simulink model "ex2"  (R2021a)
settings: Solver=VariableStepAuto  StartTime=0.0  StopTime=10.0  RelTol=1e-3
undefined symbols (not defined in the file or in its folder): B, g, I_xx, I_yy, I_zz, k, kd, l, m
settings Model: Creator=frede  LastModifiedBy=frede
settings DataIOCC: ReturnWorkspaceOutputs=off

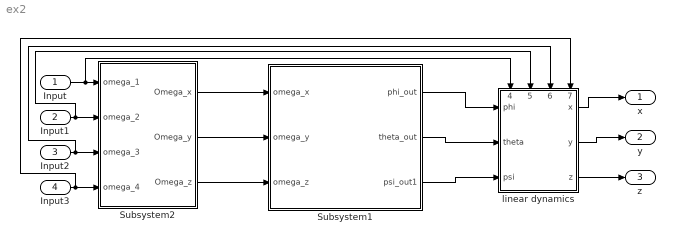
== system ex2 ==
  Input : Inport
  Input1 : Inport  Port=2
  Input2 : Inport  Port=3
  Input3 : Inport  Port=4
  Subsystem1 : Subsystem
  Subsystem2 : Subsystem
  linear dynamics : Subsystem
      settings: PortSchema="{\"entries\":[{\"content\":{\"sides\":[{\"content\":{\"connectorIds\":[\"In1\",\"In2\",\"In3\"]},\"type\":\"ConnectorPlacement.EquallySpacedRectSide\",\"uuid\":\"56efaa7c-52a2-4b92-9bf3-e77850251265\"},{\"content\":{\"connectorIds\":[\"Out1\",\"Out2\",\"Out3\"],\"side\":\"RIGHT\"},\"type\":\"ConnectorPlacement.EquallySpacedRectSide\",\"uuid\":\"60524467-1949-4cc2-aa81-2e6d1e137057\"},{\"content\":{\"connectorIds\":[\"In4\",\"In5\",\"In6\",\"In7\"],\"side\":\"TOP\"},\"type\":\"ConnectorPlacement.EquallySpacedRectSide\",\"uuid\":\"33c04961-8bd6-41a2-b762-88d931b05d2b\"},{\"content\":{\"connectorIds\":[],\"side\":\"BOTTOM\"},\"type\":\"ConnectorPlacement.EquallySpacedRectSide\",\"uuid\":\"e0b8ebeb-9596-486e-9ed8-6640ac8c0b72\"}]},\"type\":\"ConnectorPlacement.EquallySpacedConnector\",\"uuid\":\"36d70e4f-9f0c-4c3e-93dc-a7f10cedf419\"}],\"packageUris\":[\"http://schema.mathworks.com/mf0/Connector/R2020b\"],\"version\":\"1.0\"}"
  x : Outport
  y : Outport  Port=2
  z : Outport  Port=3
  wires:
  linear dynamics/1(x) -> x/1
  linear dynamics/2(y) -> y/1
  linear dynamics/3(z) -> z/1
  Subsystem1/1(phi_out) -> linear dynamics/1(phi)
  Subsystem1/3(psi_out1) -> linear dynamics/3(psi)
  Subsystem2/1(Omega_x) -> Subsystem1/1(omega_x)
  Subsystem2/2(Omega_y) -> Subsystem1/2(omega_y)
  Subsystem2/3(Omega_z) -> Subsystem1/3(omega_z)
  Subsystem1/2(theta_out) -> linear dynamics/2(theta)
  Input/1 -> linear dynamics/4(Input), Subsystem2/1(omega_1)
  Input1/1 -> Subsystem2/2(omega_2), linear dynamics/5(Input1)
  Input2/1 -> Subsystem2/3(omega_3), linear dynamics/6(Input2)
  Input3/1 -> Subsystem2/4(omega_4), linear dynamics/7(Input3)

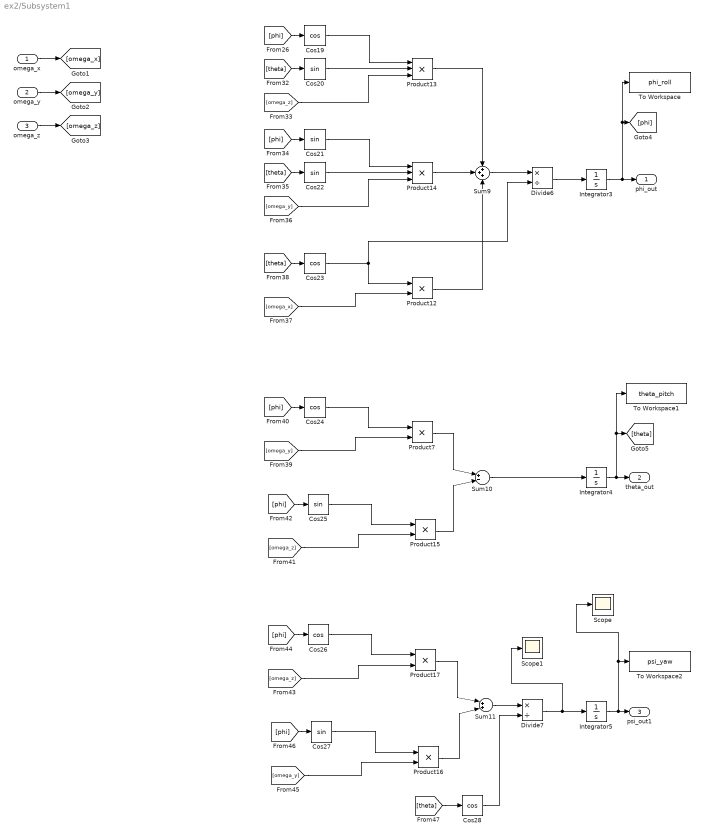
== system ex2/Subsystem1 ==
  omega_x : Inport
  omega_y : Inport  Port=2
  omega_z : Inport  Port=3
  Cos{19,23..24,26,28} (5 alike) : Trigonometry  Operator=cos
  Cos{20..22,25,27} (5 alike) : Trigonometry
  Divide6 : Product  Inputs=*/
  Divide7 : Product  Inputs=*/
  Integrator3 : Integrator
  Integrator4 : Integrator
  Integrator5 : Integrator
  Product{7,12,15..17} (5 alike) : Product
  Product13 : Product  Inputs=3
  Product14 : Product  Inputs=3
  Scope : Scope
  Scope1 : Scope
  Sum10 : Sum  Inputs=|+-|
  Sum11 : Sum  Inputs=|++|
  Sum9 : Sum  Inputs=+++
  To Workspace : ToWorkspace  VariableName=phi_roll  SaveFormat=Timeseries  SampleTime=-1
  To Workspace1 : ToWorkspace  VariableName=theta_pitch  SaveFormat=Timeseries  SampleTime=-1
  To Workspace2 : ToWorkspace  VariableName=psi_yaw  SaveFormat=Timeseries  SampleTime=-1
  phi_out : Outport
  theta_out : Outport  Port=2
  psi_out1 : Outport  Port=3
  wires:
  omega_x/1 -> [omega_x]
  omega_y/1 -> [omega_y]
  omega_z/1 -> [omega_z]
  Cos19/1 -> Product13/1
  [phi] -> Cos19/1
  Cos20/1 -> Product13/2
  [theta] -> Cos20/1
  [omega_z] -> Product13/3
  Cos22/1 -> Product14/2
  [theta] -> Cos22/1
  [phi] -> Cos21/1
  Cos21/1 -> Product14/1
  [omega_y] -> Product14/3
  [omega_x] -> Product12/2
  [theta] -> Cos23/1
  Cos23/1 -> Product12/1, Divide6/2
  Product14/1 -> Sum9/2
  Product13/1 -> Sum9/1
  Product12/1 -> Sum9/3
  Sum9/1 -> Divide6/1
  Divide6/1 -> Integrator3/1
  Integrator3/1 -> To Workspace/1, [phi], phi_out/1
  [omega_y] -> Product7/2
  Cos24/1 -> Product7/1
  [phi] -> Cos24/1
  [phi] -> Cos25/1
  Cos25/1 -> Product15/1
  [omega_z] -> Product15/2
  Product15/1 -> Sum10/2
  Product7/1 -> Sum10/1
  Sum10/1 -> Integrator4/1
  Integrator4/1 -> To Workspace1/1, [theta], theta_out/1
  Product17/1 -> Sum11/1
  [phi] -> Cos26/1
  [omega_z] -> Product17/2
  Cos27/1 -> Product16/1
  [phi] -> Cos27/1
  Integrator5/1 -> Scope/1, To Workspace2/1, psi_out1/1
  [omega_y] -> Product16/2
  Cos26/1 -> Product17/1
  Product16/1 -> Sum11/2
  Sum11/1 -> Divide7/1
  Cos28/1 -> Divide7/2
  [theta] -> Cos28/1
  Divide7/1 -> Scope1/1, Integrator5/1

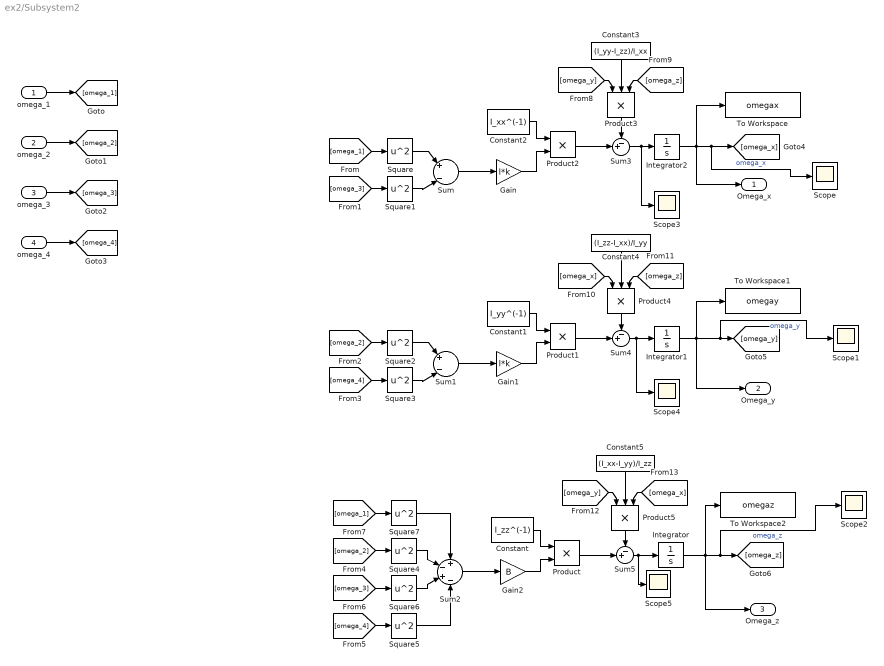
== system ex2/Subsystem2 ==
  omega_1 : Inport
  omega_2 : Inport  Port=2
  omega_3 : Inport  Port=3
  omega_4 : Inport  Port=4
  Constant : Constant  Value=I_zz^(-1)
  Constant1 : Constant  Value=I_yy^(-1)
  Constant2 : Constant  Value=I_xx^(-1)
  Constant3 : Constant  Value=(I_yy-I_zz)/I_xx
  Constant4 : Constant  Value=(I_zz-I_xx)/I_yy
  Constant5 : Constant  Value=(I_xx-I_yy)/I_zz
  Gain : Gain  Gain=l*k
  Gain1 : Gain  Gain=l*k
  Gain2 : Gain  Gain=B
  Integrator : Integrator
  Integrator1 : Integrator
  Integrator2 : Integrator
  Product : Product
  Product1 : Product
  Product2 : Product
  Product3 : Product  Inputs=3
  Product4 : Product  Inputs=3
  Product5 : Product  Inputs=3
  Scope{,1..5} (6 alike) : Scope
  Square{,1..7} (8 alike) : Math  Operator=square  SaturateOnIntegerOverflow=on
  Sum : Sum  Inputs=|+|-|
  Sum1 : Sum  Inputs=|+|-|
  Sum2 : Sum  Inputs=+-+-
  Sum3 : Sum  Inputs=-+|
  Sum4 : Sum  Inputs=-+|
  Sum5 : Sum  Inputs=-+|
  To Workspace : ToWorkspace  VariableName=omegax  SaveFormat=Timeseries  SampleTime=-1
  To Workspace1 : ToWorkspace  VariableName=omegay  SaveFormat=Timeseries  SampleTime=-1
  To Workspace2 : ToWorkspace  VariableName=omegaz  SaveFormat=Timeseries  SampleTime=-1
  Omega_x : Outport
  Omega_y : Outport  Port=2
  Omega_z : Outport  Port=3
  wires:
  omega_1/1 -> [omega_1]
  omega_2/1 -> [omega_2]
  omega_3/1 -> [omega_3]
  omega_4/1 -> [omega_4]
  [omega_1] -> Square/1
  Square/1 -> Sum/1
  [omega_3] -> Square1/1
  Square1/1 -> Sum/2
  Sum/1 -> Gain/1
  Square3/1 -> Sum1/2
  Sum1/1 -> Gain1/1
  [omega_2] -> Square2/1
  Square2/1 -> Sum1/1
  [omega_4] -> Square3/1
  Square4/1 -> Sum2/2
  Sum2/1 -> Gain2/1
  Square5/1 -> Sum2/4
  [omega_4] -> Square5/1
  [omega_2] -> Square4/1
  [omega_3] -> Square6/1
  Square6/1 -> Sum2/3
  [omega_1] -> Square7/1
  Square7/1 -> Sum2/1
  Gain2/1 -> Product/2
  Constant/1 -> Product/1
  Constant1/1 -> Product1/1
  Gain1/1 -> Product1/2
  Constant2/1 -> Product2/1
  Gain/1 -> Product2/2
  Product2/1 -> Sum3/2
  Product1/1 -> Sum4/2
  Product/1 -> Sum5/2
  Sum3/1 -> Scope3/1, Integrator2/1
  Sum4/1 -> Scope4/1, Integrator1/1
  Integrator/1 -> To Workspace2/1, Omega_z/1, Scope2/1, [omega_z]  "omega_z"
  Integrator1/1 -> To Workspace1/1, Omega_y/1, Scope1/1, [omega_y]  "omega_y"
  Integrator2/1 -> To Workspace/1, Omega_x/1, Scope/1, [omega_x]  "omega_x"
  Product3/1 -> Sum3/1
  Constant3/1 -> Product3/2
  [omega_z] -> Product3/3
  [omega_y] -> Product3/1
  Product4/1 -> Sum4/1
  [omega_x] -> Product4/1
  [omega_z] -> Product4/3
  Constant4/1 -> Product4/2
  Product5/1 -> Sum5/1
  [omega_y] -> Product5/1
  [omega_x] -> Product5/3
  Constant5/1 -> Product5/2
  Sum5/1 -> Scope5/1, Integrator/1

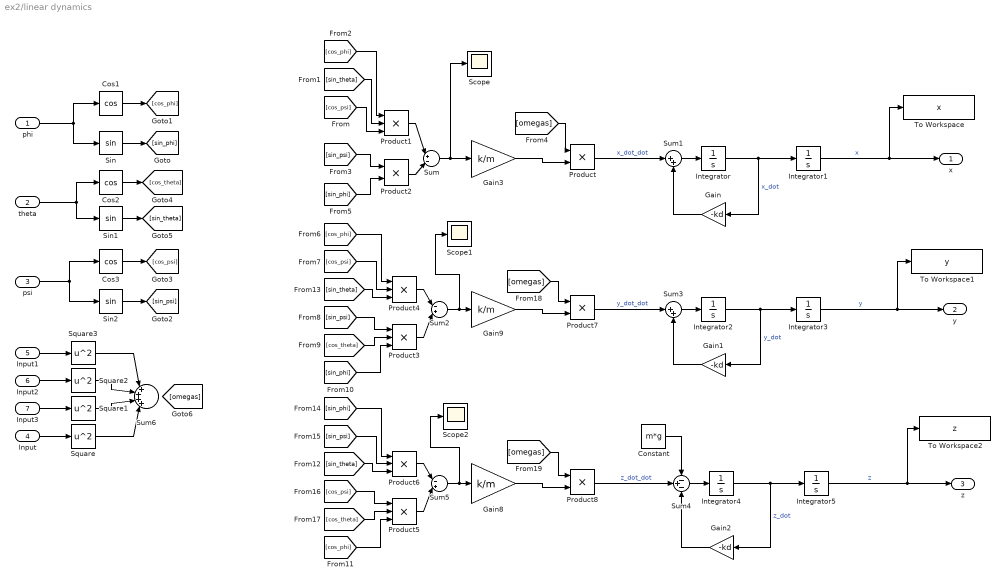
== system ex2/linear dynamics ==
  phi : Inport
  theta : Inport  Port=2
  psi : Inport  Port=3
  Input : Inport  Port=4
  Input1 : Inport  Port=5
  Input2 : Inport  Port=6
  Input3 : Inport  Port=7
  Constant : Constant  Value=m*g
  Cos1 : Trigonometry  Operator=cos
  Cos2 : Trigonometry  Operator=cos
  Cos3 : Trigonometry  Operator=cos
  Gain : Gain  Gain=-kd
  Gain1 : Gain  Gain=-kd
  Gain2 : Gain  Gain=-kd
  Gain3 : Gain  Gain=k/m
  Gain8 : Gain  Gain=k/m
  Gain9 : Gain  Gain=k/m
  Integrator{,1..5} (6 alike) : Integrator
  Product{,2,7..8} (4 alike) : Product
  Product{1,3..6} (5 alike) : Product  Inputs=3
  Scope : Scope
  Scope1 : Scope
  Scope2 : Scope
  Sin : Trigonometry
  Sin1 : Trigonometry
  Sin2 : Trigonometry
  Square{,1..3} (4 alike) : Math  Operator=square  SaturateOnIntegerOverflow=on
  Sum : Sum  Inputs=|+-|
  Sum1 : Sum  Inputs=|++
  Sum2 : Sum  Inputs=|-+|
  Sum3 : Sum  Inputs=|++
  Sum4 : Sum  Inputs=-+-
  Sum5 : Sum  Inputs=|-+|
  Sum6 : Sum  Inputs=|++++|
  To Workspace : ToWorkspace  VariableName=x  SaveFormat=Timeseries  SampleTime=-1
  To Workspace1 : ToWorkspace  VariableName=y  SaveFormat=Timeseries  SampleTime=-1
  To Workspace2 : ToWorkspace  VariableName=z  SaveFormat=Timeseries  SampleTime=-1
  x : Outport
  y : Outport  Port=2
  z : Outport  Port=3
  wires:
  Gain/1 -> Sum1/2
  Integrator5/1 -> z/1, To Workspace2/1  "z"
  [cos_phi] -> Product4/1
  Product2/1 -> Sum/2
  [sin_psi] -> Product3/1
  Sum1/1 -> Integrator/1
  Sum/1 -> Scope/1, Gain3/1
  [sin_theta] -> Product1/2
  phi/1 -> Cos1/1, Sin/1
  Gain1/1 -> Sum3/2
  Integrator3/1 -> y/1, To Workspace1/1  "y"
  [sin_psi] -> Product2/1
  Product3/1 -> Sum2/2
  Integrator2/1 -> Gain1/1, Integrator3/1  "y_dot"
  psi/1 -> Sin2/1, Cos3/1
  [cos_phi] -> Product5/3
  Cos2/1 -> [cos_theta]
  [sin_theta] -> Product6/3
  [cos_psi] -> Product1/3
  Integrator1/1 -> x/1, To Workspace/1  "x"
  Sum3/1 -> Integrator2/1
  Sum5/1 -> Scope2/1, Gain8/1
  Product/1 -> Sum1/1  "x_dot_dot"
  Integrator4/1 -> Gain2/1, Integrator5/1  "z_dot"
  [sin_phi] -> Product3/3
  [cos_psi] -> Product4/2
  Product1/1 -> Sum/1
  Cos3/1 -> [cos_psi]
  [cos_psi] -> Product5/1
  [sin_psi] -> Product6/2
  [cos_phi] -> Product1/1
  Product6/1 -> Sum5/1
  Product5/1 -> Sum5/2
  Gain3/1 -> Product/2
  Integrator/1 -> Gain/1, Integrator1/1  "x_dot"
  Sin1/1 -> [sin_theta]
  Sum2/1 -> Scope1/1, Gain9/1
  [sin_theta] -> Product4/3
  [sin_phi] -> Product6/1
  [cos_theta] -> Product5/2
  Sin2/1 -> [sin_psi]
  Cos1/1 -> [cos_phi]
  theta/1 -> Cos2/1, Sin1/1
  [cos_theta] -> Product3/2
  Sum4/1 -> Integrator4/1
  Gain2/1 -> Sum4/3
  Product4/1 -> Sum2/1
  Constant/1 -> Sum4/1
  Sin/1 -> [sin_phi]
  [sin_phi] -> Product2/2
  Input/1 -> Square/1
  Input3/1 -> Square1/1
  Input2/1 -> Square2/1
  Input1/1 -> Square3/1
  Square/1 -> Sum6/4
  Square1/1 -> Sum6/3
  Square2/1 -> Sum6/2
  Square3/1 -> Sum6/1
  [omegas] -> Product/1
  [omegas] -> Product7/1
  Product7/1 -> Sum3/1  "y_dot_dot"
  Gain9/1 -> Product7/2
  [omegas] -> Product8/1
  Gain8/1 -> Product8/2
  Product8/1 -> Sum4/2  "z_dot_dot"
